simulink library "INP_ERR"  (R2024b)
settings: Solver=VariableStepAuto  StartTime=0.0  StopTime=10.0  RelTol=1e-3
settings Model: Creator=blatak  LastModifiedBy=jmbsp

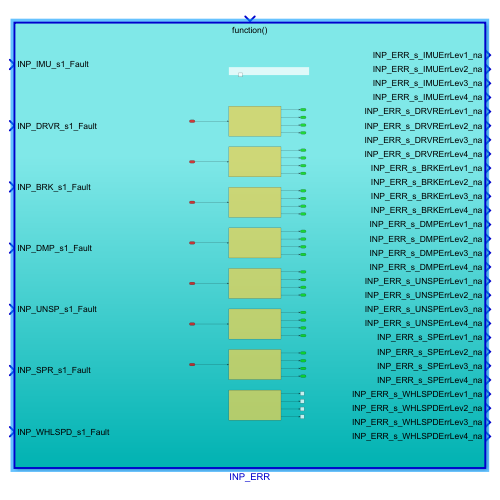
[thumbnail: Simulink's stored preview of the top-level diagram]
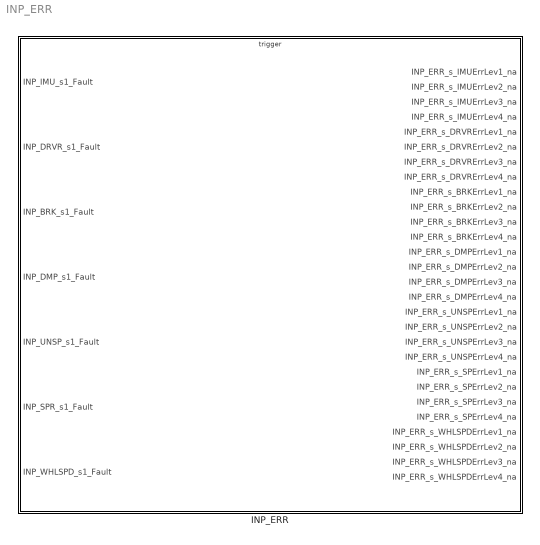
== system INP_ERR ==
  INP_ERR : Subsystem  TreatAsAtomicUnit=on

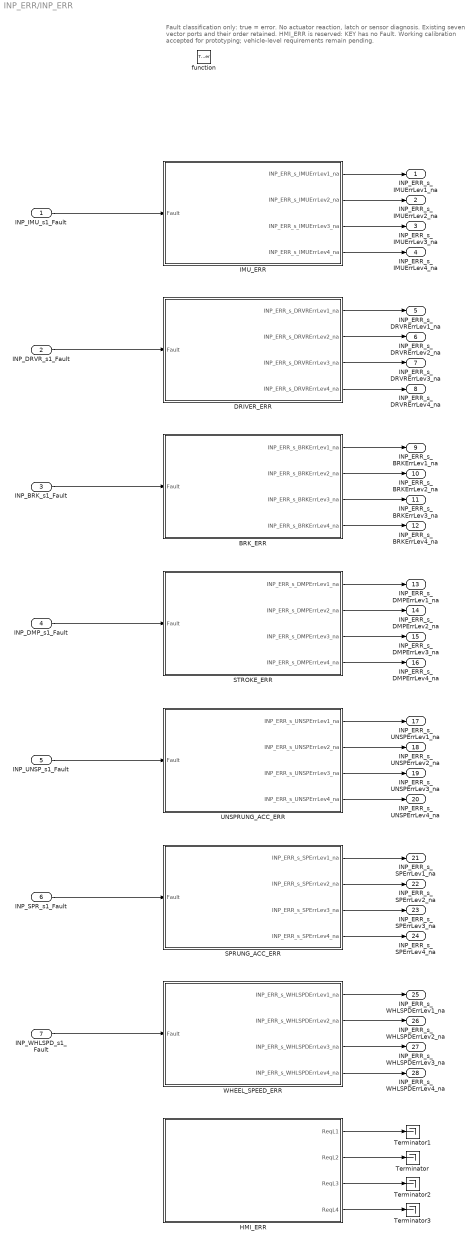
== system INP_ERR/INP_ERR ==
  note: Fault classification only: true = error. No actuator reaction, latch or sensor diagnosis.
      | Existing seven vector ports and their order retained. HMI_ERR is reserved: KEY has no Fault.
      | Working calibration accepted for prototyping; vehicle-level requirements remain pending.
  INP_IMU_s1_Fault : Inport  OutDataTypeStr=boolean  PortDimensions=6
  INP_DRVR_s1_Fault : Inport  Port=2  OutDataTypeStr=boolean  PortDimensions=2
  INP_BRK_s1_Fault : Inport  Port=3  OutDataTypeStr=boolean  PortDimensions=2
  INP_DMP_s1_Fault : Inport  Port=4  OutDataTypeStr=boolean  PortDimensions=8
  INP_UNSP_s1_Fault : Inport  Port=5  OutDataTypeStr=boolean  PortDimensions=4
  INP_SPR_s1_Fault : Inport  Port=6  OutDataTypeStr=boolean  PortDimensions=4
  INP_WHLSPD_s1_Fault : Inport  Port=7  OutDataTypeStr=boolean  PortDimensions=4
  function : TriggerPort  TriggerType=function-call  VariantControl=(inherit)
  BRK_ERR : Subsystem
  DRIVER_ERR : Subsystem
  HMI_ERR : Subsystem
  IMU_ERR : Subsystem
  SPRUNG_ACC_ERR : Subsystem
  STROKE_ERR : Subsystem
  Terminator{,1..3} (4 alike) : Terminator
  UNSPRUNG_ACC_ERR : Subsystem
  WHEEL_SPEED_ERR : Subsystem
  INP_ERR_s_IMUErrLev1_na : Outport
  INP_ERR_s_IMUErrLev2_na : Outport  Port=2
  INP_ERR_s_IMUErrLev3_na : Outport  Port=3
  INP_ERR_s_IMUErrLev4_na : Outport  Port=4
  INP_ERR_s_DRVRErrLev1_na : Outport  Port=5
  INP_ERR_s_DRVRErrLev2_na : Outport  Port=6
  INP_ERR_s_DRVRErrLev3_na : Outport  Port=7
  INP_ERR_s_DRVRErrLev4_na : Outport  Port=8
  INP_ERR_s_BRKErrLev1_na : Outport  Port=9
  INP_ERR_s_BRKErrLev2_na : Outport  Port=10
  INP_ERR_s_BRKErrLev3_na : Outport  Port=11
  INP_ERR_s_BRKErrLev4_na : Outport  Port=12
  INP_ERR_s_DMPErrLev1_na : Outport  Port=13
  INP_ERR_s_DMPErrLev2_na : Outport  Port=14
  INP_ERR_s_DMPErrLev3_na : Outport  Port=15
  INP_ERR_s_DMPErrLev4_na : Outport  Port=16
  INP_ERR_s_UNSPErrLev1_na : Outport  Port=17
  INP_ERR_s_UNSPErrLev2_na : Outport  Port=18
  INP_ERR_s_UNSPErrLev3_na : Outport  Port=19
  INP_ERR_s_UNSPErrLev4_na : Outport  Port=20
  INP_ERR_s_SPErrLev1_na : Outport  Port=21
  INP_ERR_s_SPErrLev2_na : Outport  Port=22
  INP_ERR_s_SPErrLev3_na : Outport  Port=23
  INP_ERR_s_SPErrLev4_na : Outport  Port=24
  INP_ERR_s_WHLSPDErrLev1_na : Outport  Port=25
  INP_ERR_s_WHLSPDErrLev2_na : Outport  Port=26
  INP_ERR_s_WHLSPDErrLev3_na : Outport  Port=27
  INP_ERR_s_WHLSPDErrLev4_na : Outport  Port=28
  wires:
  INP_IMU_s1_Fault/1 -> IMU_ERR/1(Fault)
  INP_DRVR_s1_Fault/1 -> DRIVER_ERR/1(Fault)
  INP_BRK_s1_Fault/1 -> BRK_ERR/1(Fault)
  INP_DMP_s1_Fault/1 -> STROKE_ERR/1(Fault)
  INP_UNSP_s1_Fault/1 -> UNSPRUNG_ACC_ERR/1(Fault)
  INP_SPR_s1_Fault/1 -> SPRUNG_ACC_ERR/1(Fault)
  INP_WHLSPD_s1_Fault/1 -> WHEEL_SPEED_ERR/1(Fault)
  IMU_ERR/1(INP_ERR_s_IMUErrLev1_na) -> INP_ERR_s_IMUErrLev1_na/1
  IMU_ERR/2(INP_ERR_s_IMUErrLev2_na) -> INP_ERR_s_IMUErrLev2_na/1
  IMU_ERR/3(INP_ERR_s_IMUErrLev3_na) -> INP_ERR_s_IMUErrLev3_na/1
  IMU_ERR/4(INP_ERR_s_IMUErrLev4_na) -> INP_ERR_s_IMUErrLev4_na/1
  DRIVER_ERR/1(INP_ERR_s_DRVRErrLev1_na) -> INP_ERR_s_DRVRErrLev1_na/1
  DRIVER_ERR/2(INP_ERR_s_DRVRErrLev2_na) -> INP_ERR_s_DRVRErrLev2_na/1
  DRIVER_ERR/3(INP_ERR_s_DRVRErrLev3_na) -> INP_ERR_s_DRVRErrLev3_na/1
  DRIVER_ERR/4(INP_ERR_s_DRVRErrLev4_na) -> INP_ERR_s_DRVRErrLev4_na/1
  HMI_ERR/1(ReqL1) -> Terminator1/1
  HMI_ERR/2(ReqL2) -> Terminator/1
  HMI_ERR/3(ReqL3) -> Terminator2/1
  HMI_ERR/4(ReqL4) -> Terminator3/1
  BRK_ERR/1(INP_ERR_s_BRKErrLev1_na) -> INP_ERR_s_BRKErrLev1_na/1
  BRK_ERR/2(INP_ERR_s_BRKErrLev2_na) -> INP_ERR_s_BRKErrLev2_na/1
  BRK_ERR/3(INP_ERR_s_BRKErrLev3_na) -> INP_ERR_s_BRKErrLev3_na/1
  BRK_ERR/4(INP_ERR_s_BRKErrLev4_na) -> INP_ERR_s_BRKErrLev4_na/1
  STROKE_ERR/1(INP_ERR_s_DMPErrLev1_na) -> INP_ERR_s_DMPErrLev1_na/1
  STROKE_ERR/2(INP_ERR_s_DMPErrLev2_na) -> INP_ERR_s_DMPErrLev2_na/1
  STROKE_ERR/3(INP_ERR_s_DMPErrLev3_na) -> INP_ERR_s_DMPErrLev3_na/1
  STROKE_ERR/4(INP_ERR_s_DMPErrLev4_na) -> INP_ERR_s_DMPErrLev4_na/1
  UNSPRUNG_ACC_ERR/1(INP_ERR_s_UNSPErrLev1_na) -> INP_ERR_s_UNSPErrLev1_na/1
  UNSPRUNG_ACC_ERR/2(INP_ERR_s_UNSPErrLev2_na) -> INP_ERR_s_UNSPErrLev2_na/1
  UNSPRUNG_ACC_ERR/3(INP_ERR_s_UNSPErrLev3_na) -> INP_ERR_s_UNSPErrLev3_na/1
  UNSPRUNG_ACC_ERR/4(INP_ERR_s_UNSPErrLev4_na) -> INP_ERR_s_UNSPErrLev4_na/1
  SPRUNG_ACC_ERR/1(INP_ERR_s_SPErrLev1_na) -> INP_ERR_s_SPErrLev1_na/1
  SPRUNG_ACC_ERR/2(INP_ERR_s_SPErrLev2_na) -> INP_ERR_s_SPErrLev2_na/1
  SPRUNG_ACC_ERR/3(INP_ERR_s_SPErrLev3_na) -> INP_ERR_s_SPErrLev3_na/1
  SPRUNG_ACC_ERR/4(INP_ERR_s_SPErrLev4_na) -> INP_ERR_s_SPErrLev4_na/1
  WHEEL_SPEED_ERR/1(INP_ERR_s_WHLSPDErrLev1_na) -> INP_ERR_s_WHLSPDErrLev1_na/1
  WHEEL_SPEED_ERR/2(INP_ERR_s_WHLSPDErrLev2_na) -> INP_ERR_s_WHLSPDErrLev2_na/1
  WHEEL_SPEED_ERR/3(INP_ERR_s_WHLSPDErrLev3_na) -> INP_ERR_s_WHLSPDErrLev3_na/1
  WHEEL_SPEED_ERR/4(INP_ERR_s_WHLSPDErrLev4_na) -> INP_ERR_s_WHLSPDErrLev4_na/1

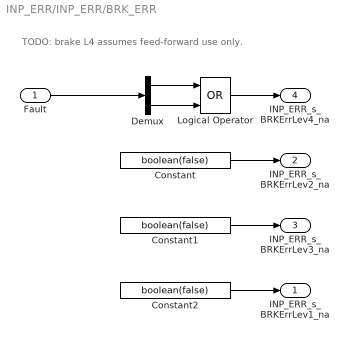
== system INP_ERR/INP_ERR/BRK_ERR ==
  note: TODO: brake L4 assumes feed-forward use only.
  Fault : Inport  OutDataTypeStr=boolean  PortDimensions=2
  Constant : Constant  Value=boolean(false)
  Constant1 : Constant  Value=boolean(false)
  Constant2 : Constant  Value=boolean(false)
  Demux : Demux  Outputs=2
  Logical Operator : Logic  Operator=OR  AllPortsSameDT=off  OutDataTypeStr=boolean
  INP_ERR_s_BRKErrLev1_na : Outport  OutDataTypeStr=boolean
  INP_ERR_s_BRKErrLev2_na : Outport  Port=2  OutDataTypeStr=boolean
  INP_ERR_s_BRKErrLev3_na : Outport  Port=3  OutDataTypeStr=boolean
  INP_ERR_s_BRKErrLev4_na : Outport  Port=4  OutDataTypeStr=boolean
  wires:
  Fault/1 -> Demux/1
  Constant1/1 -> INP_ERR_s_BRKErrLev3_na/1
  Logical Operator/1 -> INP_ERR_s_BRKErrLev4_na/1
  Constant2/1 -> INP_ERR_s_BRKErrLev1_na/1
  Constant/1 -> INP_ERR_s_BRKErrLev2_na/1
  Demux/1 -> Logical Operator/1
  Demux/2 -> Logical Operator/2

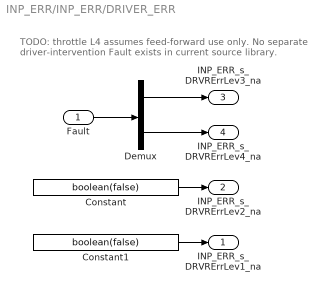
== system INP_ERR/INP_ERR/DRIVER_ERR ==
  note: TODO: throttle L4 assumes feed-forward use only.
      | No separate driver-intervention Fault exists in current source library.
  Fault : Inport  OutDataTypeStr=boolean  PortDimensions=2
  Constant : Constant  Value=boolean(false)
  Constant1 : Constant  Value=boolean(false)
  Demux : Demux  Outputs=2
  INP_ERR_s_DRVRErrLev1_na : Outport  OutDataTypeStr=boolean
  INP_ERR_s_DRVRErrLev2_na : Outport  Port=2  OutDataTypeStr=boolean
  INP_ERR_s_DRVRErrLev3_na : Outport  Port=3  OutDataTypeStr=boolean
  INP_ERR_s_DRVRErrLev4_na : Outport  Port=4  OutDataTypeStr=boolean
  wires:
  Fault/1 -> Demux/1
  Demux/1 -> INP_ERR_s_DRVRErrLev3_na/1
  Demux/2 -> INP_ERR_s_DRVRErrLev4_na/1
  Constant/1 -> INP_ERR_s_DRVRErrLev2_na/1
  Constant1/1 -> INP_ERR_s_DRVRErrLev1_na/1

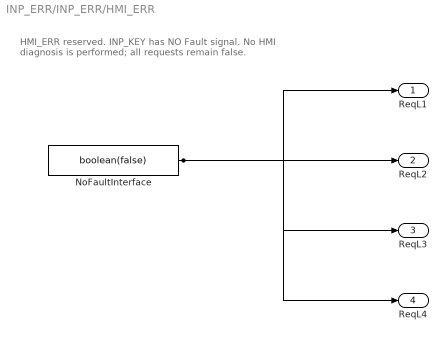
== system INP_ERR/INP_ERR/HMI_ERR ==
  note: HMI_ERR reserved. INP_KEY has NO Fault signal.
      | No HMI diagnosis is performed; all requests remain false.
  NoFaultInterface : Constant  Value=boolean(false)
  ReqL1 : Outport  OutDataTypeStr=boolean
  ReqL2 : Outport  Port=2  OutDataTypeStr=boolean
  ReqL3 : Outport  Port=3  OutDataTypeStr=boolean
  ReqL4 : Outport  Port=4  OutDataTypeStr=boolean
  wires:
  NoFaultInterface/1 -> ReqL1/1, ReqL2/1, ReqL3/1, ReqL4/1

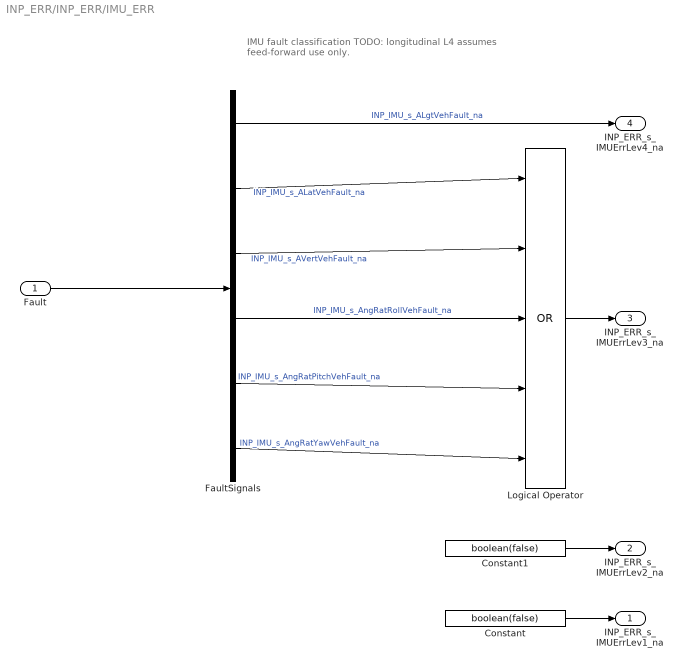
== system INP_ERR/INP_ERR/IMU_ERR ==
  note: IMU fault classification
      | TODO: longitudinal L4 assumes feed-forward use only.
  Fault : Inport  OutDataTypeStr=boolean  PortDimensions=6
  Constant : Constant  Value=boolean(false)
  Constant1 : Constant  Value=boolean(false)
  FaultSignals : Demux  Outputs=6
  Logical Operator : Logic  Operator=OR  Inputs=5  AllPortsSameDT=off  OutDataTypeStr=boolean
  INP_ERR_s_IMUErrLev1_na : Outport  OutDataTypeStr=boolean
  INP_ERR_s_IMUErrLev2_na : Outport  Port=2  OutDataTypeStr=boolean
  INP_ERR_s_IMUErrLev3_na : Outport  Port=3  OutDataTypeStr=boolean
  INP_ERR_s_IMUErrLev4_na : Outport  Port=4  OutDataTypeStr=boolean
  wires:
  Fault/1 -> FaultSignals/1
  FaultSignals/3 -> Logical Operator/2  "INP_IMU_s_AVertVehFault_na"
  FaultSignals/1 -> INP_ERR_s_IMUErrLev4_na/1  "INP_IMU_s_ALgtVehFault_na"
  FaultSignals/2 -> Logical Operator/1  "INP_IMU_s_ALatVehFault_na"
  FaultSignals/4 -> Logical Operator/3  "INP_IMU_s_AngRatRollVehFault_na"
  FaultSignals/5 -> Logical Operator/4  "INP_IMU_s_AngRatPitchVehFault_na"
  FaultSignals/6 -> Logical Operator/5  "INP_IMU_s_AngRatYawVehFault_na"
  Constant1/1 -> INP_ERR_s_IMUErrLev2_na/1
  Constant/1 -> INP_ERR_s_IMUErrLev1_na/1
  Logical Operator/1 -> INP_ERR_s_IMUErrLev3_na/1

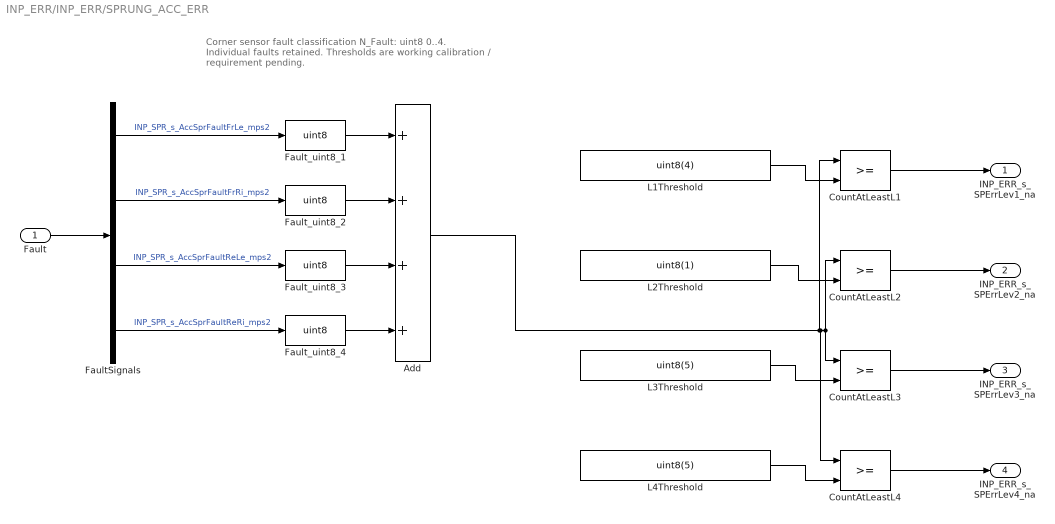
== system INP_ERR/INP_ERR/SPRUNG_ACC_ERR ==
  note: Corner sensor fault classification
      | N_Fault: uint8 0..4. Individual faults retained.
      | Thresholds are working calibration / requirement pending.
  Fault : Inport  OutDataTypeStr=boolean  PortDimensions=4
  Add : Sum  Inputs=++++
  CountAtLeastL{1..4} (4 alike) : RelationalOperator  OutDataTypeStr=boolean  RndMeth=Simplest  InputSameDT=off
  FaultSignals : Demux
  Fault_uint8_{1..4} (4 alike) : DataTypeConversion  OutDataTypeStr=uint8  SaturateOnIntegerOverflow=off  RndMeth=Floor
  L1Threshold : Constant  Description=|  Value=uint8(4)
      | INP_ERR_p_SPRUNG_ACCL1Count_na
      | TODO minimum faulty corners for SPRUNG_ACC_ERR L1; 5 disables
  L2Threshold : Constant  Description=|  Value=uint8(1)
      | INP_ERR_p_SPRUNG_ACCL2Count_na
      | TODO minimum faulty corners for SPRUNG_ACC_ERR L2; 5 disables
  L3Threshold : Constant  Description=|  Value=uint8(5)
      | INP_ERR_p_SPRUNG_ACCL3Count_na
      | TODO minimum faulty corners for SPRUNG_ACC_ERR L3; 5 disables
  L4Threshold : Constant  Description=|  Value=uint8(5)
      | INP_ERR_p_SPRUNG_ACCL4Count_na
      | TODO minimum faulty corners for SPRUNG_ACC_ERR L4; 5 disables
  INP_ERR_s_SPErrLev1_na : Outport  OutDataTypeStr=boolean
  INP_ERR_s_SPErrLev2_na : Outport  Port=2  OutDataTypeStr=boolean
  INP_ERR_s_SPErrLev3_na : Outport  Port=3  OutDataTypeStr=boolean
  INP_ERR_s_SPErrLev4_na : Outport  Port=4  OutDataTypeStr=boolean
  wires:
  Fault/1 -> FaultSignals/1
  FaultSignals/1 -> Fault_uint8_1/1  "INP_SPR_s_AccSprFaultFrLe_mps2"
  FaultSignals/2 -> Fault_uint8_2/1  "INP_SPR_s_AccSprFaultFrRi_mps2"
  FaultSignals/3 -> Fault_uint8_3/1  "INP_SPR_s_AccSprFaultReLe_mps2"
  FaultSignals/4 -> Fault_uint8_4/1  "INP_SPR_s_AccSprFaultReRi_mps2"
  Add/1 -> CountAtLeastL2/1, CountAtLeastL3/1, CountAtLeastL4/1, CountAtLeastL1/1
  L1Threshold/1 -> CountAtLeastL1/2
  CountAtLeastL1/1 -> INP_ERR_s_SPErrLev1_na/1
  L2Threshold/1 -> CountAtLeastL2/2
  CountAtLeastL2/1 -> INP_ERR_s_SPErrLev2_na/1
  L3Threshold/1 -> CountAtLeastL3/2
  CountAtLeastL3/1 -> INP_ERR_s_SPErrLev3_na/1
  L4Threshold/1 -> CountAtLeastL4/2
  CountAtLeastL4/1 -> INP_ERR_s_SPErrLev4_na/1
  Fault_uint8_1/1 -> Add/1
  Fault_uint8_2/1 -> Add/2
  Fault_uint8_3/1 -> Add/3
  Fault_uint8_4/1 -> Add/4

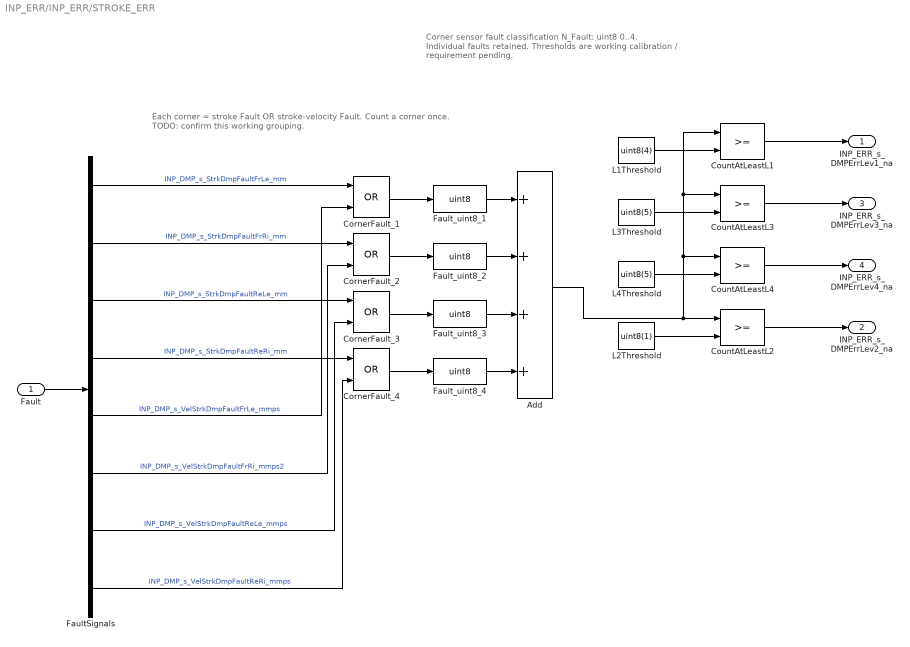
== system INP_ERR/INP_ERR/STROKE_ERR ==
  note: Each corner = stroke Fault OR stroke-velocity Fault. Count a corner once.
      | TODO: confirm this working grouping.
  note: Corner sensor fault classification
      | N_Fault: uint8 0..4. Individual faults retained.
      | Thresholds are working calibration / requirement pending.
  Fault : Inport  OutDataTypeStr=boolean  PortDimensions=8
  Add : Sum  Inputs=++++
  CornerFault_{1..4} (4 alike) : Logic  Operator=OR  AllPortsSameDT=off  OutDataTypeStr=boolean
  CountAtLeastL{1..4} (4 alike) : RelationalOperator  OutDataTypeStr=boolean  RndMeth=Simplest  InputSameDT=off
  FaultSignals : Demux  Outputs=8
  Fault_uint8_{1..4} (4 alike) : DataTypeConversion  OutDataTypeStr=uint8  SaturateOnIntegerOverflow=off  RndMeth=Floor
  L1Threshold : Constant  Description=|  Value=uint8(4)
      | INP_ERR_p_STROKEL1Count_na
      | TODO minimum faulty corners for STROKE_ERR L1; 5 disables
  L2Threshold : Constant  Description=|  Value=uint8(1)
      | INP_ERR_p_STROKEL2Count_na
      | TODO minimum faulty corners for STROKE_ERR L2; 5 disables
  L3Threshold : Constant  Description=|  Value=uint8(5)
      | INP_ERR_p_STROKEL3Count_na
      | TODO minimum faulty corners for STROKE_ERR L3; 5 disables
  L4Threshold : Constant  Description=|  Value=uint8(5)
      | INP_ERR_p_STROKEL4Count_na
      | TODO minimum faulty corners for STROKE_ERR L4; 5 disables
  INP_ERR_s_DMPErrLev1_na : Outport  OutDataTypeStr=boolean
  INP_ERR_s_DMPErrLev2_na : Outport  Port=2  OutDataTypeStr=boolean
  INP_ERR_s_DMPErrLev3_na : Outport  Port=3  OutDataTypeStr=boolean
  INP_ERR_s_DMPErrLev4_na : Outport  Port=4  OutDataTypeStr=boolean
  wires:
  CountAtLeastL2/1 -> INP_ERR_s_DMPErrLev2_na/1
  CornerFault_2/1 -> Fault_uint8_2/1
  FaultSignals/6 -> CornerFault_2/2  "INP_DMP_s_VelStrkDmpFaultFrRi_mmps2"
  FaultSignals/4 -> CornerFault_4/1  "INP_DMP_s_StrkDmpFaultReRi_mm"
  CountAtLeastL1/1 -> INP_ERR_s_DMPErrLev1_na/1
  CornerFault_1/1 -> Fault_uint8_1/1
  FaultSignals/2 -> CornerFault_2/1  "INP_DMP_s_StrkDmpFaultFrRi_mm"
  CountAtLeastL4/1 -> INP_ERR_s_DMPErrLev4_na/1
  CornerFault_4/1 -> Fault_uint8_4/1
  Fault/1 -> FaultSignals/1
  FaultSignals/7 -> CornerFault_3/2  "INP_DMP_s_VelStrkDmpFaultReLe_mmps"
  FaultSignals/5 -> CornerFault_1/2  "INP_DMP_s_VelStrkDmpFaultFrLe_mmps"
  FaultSignals/3 -> CornerFault_3/1  "INP_DMP_s_StrkDmpFaultReLe_mm"
  FaultSignals/1 -> CornerFault_1/1  "INP_DMP_s_StrkDmpFaultFrLe_mm"
  FaultSignals/8 -> CornerFault_4/2  "INP_DMP_s_VelStrkDmpFaultReRi_mmps"
  CountAtLeastL3/1 -> INP_ERR_s_DMPErrLev3_na/1
  CornerFault_3/1 -> Fault_uint8_3/1
  L1Threshold/1 -> CountAtLeastL1/2
  L3Threshold/1 -> CountAtLeastL3/2
  L4Threshold/1 -> CountAtLeastL4/2
  L2Threshold/1 -> CountAtLeastL2/2
  Fault_uint8_4/1 -> Add/4
  Fault_uint8_3/1 -> Add/3
  Fault_uint8_2/1 -> Add/2
  Fault_uint8_1/1 -> Add/1
  Add/1 -> CountAtLeastL4/1, CountAtLeastL3/1, CountAtLeastL1/1, CountAtLeastL2/1

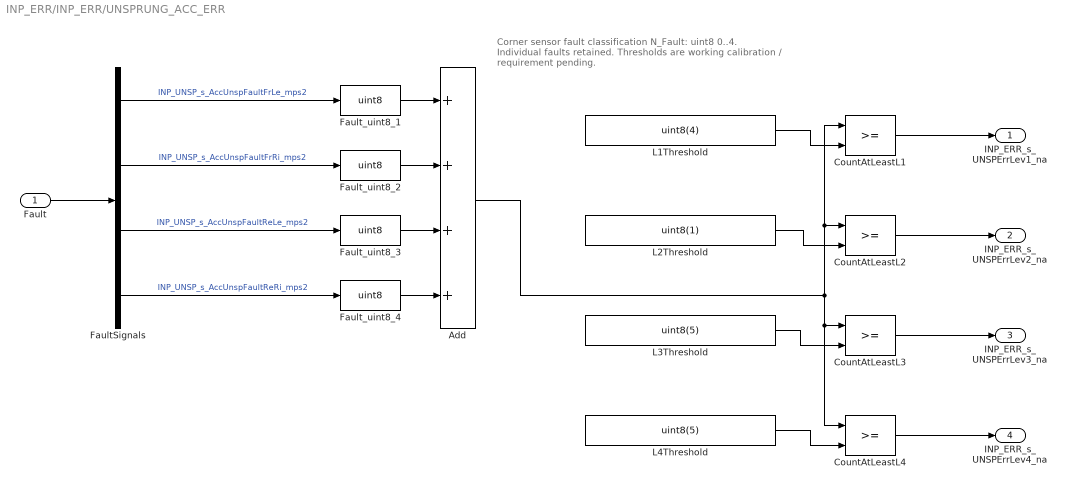
== system INP_ERR/INP_ERR/UNSPRUNG_ACC_ERR ==
  note: Corner sensor fault classification
      | N_Fault: uint8 0..4. Individual faults retained.
      | Thresholds are working calibration / requirement pending.
  Fault : Inport  OutDataTypeStr=boolean  PortDimensions=4
  Add : Sum  Inputs=++++
  CountAtLeastL{1..4} (4 alike) : RelationalOperator  OutDataTypeStr=boolean  RndMeth=Simplest  InputSameDT=off
  FaultSignals : Demux
  Fault_uint8_{1..4} (4 alike) : DataTypeConversion  OutDataTypeStr=uint8  SaturateOnIntegerOverflow=off  RndMeth=Floor
  L1Threshold : Constant  Description=|  Value=uint8(4)
      | INP_ERR_p_UNSPRUNG_ACCL1Count_na
      | TODO minimum faulty corners for UNSPRUNG_ACC_ERR L1; 5 disables
  L2Threshold : Constant  Description=|  Value=uint8(1)
      | INP_ERR_p_UNSPRUNG_ACCL2Count_na
      | TODO minimum faulty corners for UNSPRUNG_ACC_ERR L2; 5 disables
  L3Threshold : Constant  Description=|  Value=uint8(5)
      | INP_ERR_p_UNSPRUNG_ACCL3Count_na
      | TODO minimum faulty corners for UNSPRUNG_ACC_ERR L3; 5 disables
  L4Threshold : Constant  Description=|  Value=uint8(5)
      | INP_ERR_p_UNSPRUNG_ACCL4Count_na
      | TODO minimum faulty corners for UNSPRUNG_ACC_ERR L4; 5 disables
  INP_ERR_s_UNSPErrLev1_na : Outport  OutDataTypeStr=boolean
  INP_ERR_s_UNSPErrLev2_na : Outport  Port=2  OutDataTypeStr=boolean
  INP_ERR_s_UNSPErrLev3_na : Outport  Port=3  OutDataTypeStr=boolean
  INP_ERR_s_UNSPErrLev4_na : Outport  Port=4  OutDataTypeStr=boolean
  wires:
  Fault/1 -> FaultSignals/1
  FaultSignals/1 -> Fault_uint8_1/1  "INP_UNSP_s_AccUnspFaultFrLe_mps2"
  FaultSignals/2 -> Fault_uint8_2/1  "INP_UNSP_s_AccUnspFaultFrRi_mps2"
  FaultSignals/3 -> Fault_uint8_3/1  "INP_UNSP_s_AccUnspFaultReLe_mps2"
  FaultSignals/4 -> Fault_uint8_4/1  "INP_UNSP_s_AccUnspFaultReRi_mps2"
  Add/1 -> CountAtLeastL4/1, CountAtLeastL3/1, CountAtLeastL2/1, CountAtLeastL1/1
  L1Threshold/1 -> CountAtLeastL1/2
  CountAtLeastL1/1 -> INP_ERR_s_UNSPErrLev1_na/1
  L2Threshold/1 -> CountAtLeastL2/2
  CountAtLeastL2/1 -> INP_ERR_s_UNSPErrLev2_na/1
  L3Threshold/1 -> CountAtLeastL3/2
  CountAtLeastL3/1 -> INP_ERR_s_UNSPErrLev3_na/1
  L4Threshold/1 -> CountAtLeastL4/2
  CountAtLeastL4/1 -> INP_ERR_s_UNSPErrLev4_na/1
  Fault_uint8_1/1 -> Add/1
  Fault_uint8_2/1 -> Add/2
  Fault_uint8_3/1 -> Add/3
  Fault_uint8_4/1 -> Add/4

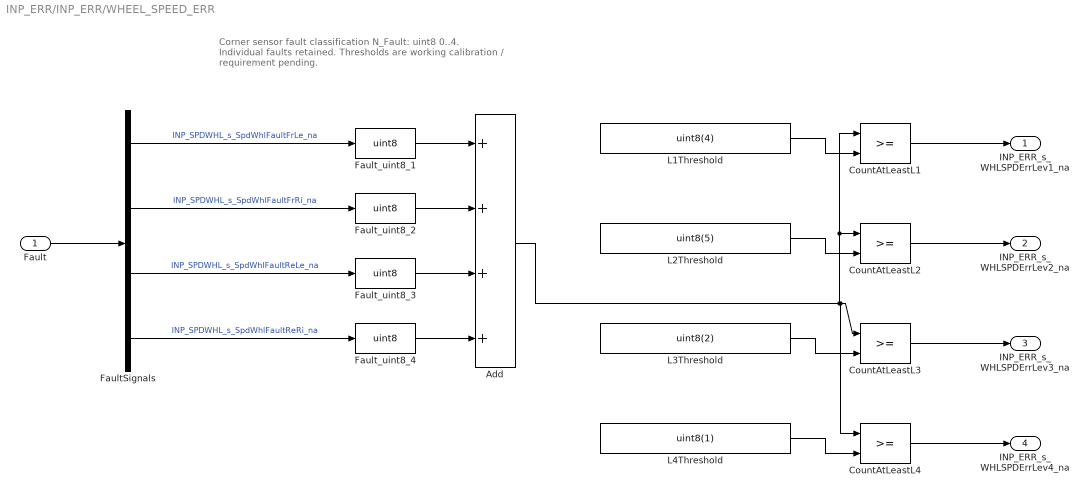
== system INP_ERR/INP_ERR/WHEEL_SPEED_ERR ==
  note: Corner sensor fault classification
      | N_Fault: uint8 0..4. Individual faults retained.
      | Thresholds are working calibration / requirement pending.
  Fault : Inport  OutDataTypeStr=boolean  PortDimensions=4
  Add : Sum  Inputs=++++
  CountAtLeastL{1..4} (4 alike) : RelationalOperator  OutDataTypeStr=boolean  RndMeth=Simplest  InputSameDT=off
  FaultSignals : Demux
  Fault_uint8_{1..4} (4 alike) : DataTypeConversion  OutDataTypeStr=uint8  SaturateOnIntegerOverflow=off  RndMeth=Floor
  L1Threshold : Constant  Description=|  Value=uint8(4)
      | INP_ERR_p_WHEEL_SPEEDL1Count_na
      | TODO minimum faulty corners for WHEEL_SPEED_ERR L1; 5 disables
  L2Threshold : Constant  Description=|  Value=uint8(5)
      | INP_ERR_p_WHEEL_SPEEDL2Count_na
      | TODO minimum faulty corners for WHEEL_SPEED_ERR L2; 5 disables
  L3Threshold : Constant  Description=|  Value=uint8(2)
      | INP_ERR_p_WHEEL_SPEEDL3Count_na
      | TODO minimum faulty corners for WHEEL_SPEED_ERR L3; 5 disables
  L4Threshold : Constant  Description=|  Value=uint8(1)
      | INP_ERR_p_WHEEL_SPEEDL4Count_na
      | TODO minimum faulty corners for WHEEL_SPEED_ERR L4; 5 disables
  INP_ERR_s_WHLSPDErrLev1_na : Outport  OutDataTypeStr=boolean
  INP_ERR_s_WHLSPDErrLev2_na : Outport  Port=2  OutDataTypeStr=boolean
  INP_ERR_s_WHLSPDErrLev3_na : Outport  Port=3  OutDataTypeStr=boolean
  INP_ERR_s_WHLSPDErrLev4_na : Outport  Port=4  OutDataTypeStr=boolean
  wires:
  Fault/1 -> FaultSignals/1
  FaultSignals/1 -> Fault_uint8_1/1  "INP_SPDWHL_s_SpdWhlFaultFrLe_na"
  Fault_uint8_1/1 -> Add/1
  FaultSignals/2 -> Fault_uint8_2/1  "INP_SPDWHL_s_SpdWhlFaultFrRi_na"
  Fault_uint8_2/1 -> Add/2
  FaultSignals/3 -> Fault_uint8_3/1  "INP_SPDWHL_s_SpdWhlFaultReLe_na"
  Fault_uint8_3/1 -> Add/3
  FaultSignals/4 -> Fault_uint8_4/1  "INP_SPDWHL_s_SpdWhlFaultReRi_na"
  Fault_uint8_4/1 -> Add/4
  Add/1 -> CountAtLeastL3/1, CountAtLeastL4/1, CountAtLeastL1/1, CountAtLeastL2/1
  L1Threshold/1 -> CountAtLeastL1/2
  CountAtLeastL1/1 -> INP_ERR_s_WHLSPDErrLev1_na/1
  L2Threshold/1 -> CountAtLeastL2/2
  CountAtLeastL2/1 -> INP_ERR_s_WHLSPDErrLev2_na/1
  L3Threshold/1 -> CountAtLeastL3/2
  CountAtLeastL3/1 -> INP_ERR_s_WHLSPDErrLev3_na/1
  L4Threshold/1 -> CountAtLeastL4/2
  CountAtLeastL4/1 -> INP_ERR_s_WHLSPDErrLev4_na/1
